simulink model "simulinkOSC_test"  (R2018b)
settings: Solver=FixedStepDiscrete  StartTime=0.0  StopTime=inf  FixedStep=0.01  RelTol=1e-3  EnableMultiTasking=on
model workspace (MAT data in the model file):
  gtest = 0
settings Model: Creator=Ulysses  LastModifiedBy=Ulysses
settings DataIOCC: LimitDataPoints=on  SaveFormat=Array
settings OptimizationCC: LifeSpan=inf
settings DebuggingCC: SolverPrmCheckMsg=warning  AllowSymbolicDim=off  SFUnexpectedBacktrackingDiag=warning  SFNoUnconditionalDefaultTransitionDiag=warning
settings HardwareCC: ProdBitPerPointer=32  ProdBitPerSizeT=32  ProdBitPerPtrDiffT=32  ProdLargestAtomicFloat=None  ProdIntDivRoundTo=Undefined  ProdEndianess=Unspecified  ProdWordSize=32  ProdHWDeviceType=32-bit Generic
settings ModelReferenceCC: PropagateSignalLabelsOutOfModel=off
settings SFSimCC: SimUseLocalCustomCode=off
settings RTWCC: RTWUseLocalCustomCode=off  TargetLang=C++
settings CodeAppCC: StateflowObjectComments=on
settings GRTTargetCC: TargetLangStandard=C89/C90 (ANSI)  GeneratePreprocessorConditionals=Disable all  MultiInstanceERTCode=on  CodeInterfacePackaging=C++ class
settings ConfigComp: CovMetricSettings=dw  CovHtmlReporting=on  CovSaveCumulativeToWorkspaceVar=on  CovSaveSingleToWorkspaceVar=on  CovExternalEMLEnable=off  CovSFcnEnable=off

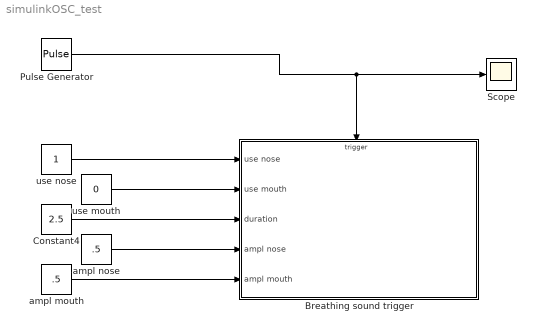
== system simulinkOSC_test ==
  Breathing sound trigger : Subsystem
  Constant4 : Constant  Value=2.5
  Pulse Generator : DiscretePulseGenerator  PulseType=Time based  Period=20000  PulseWidth=50
  Scope : Scope
  ampl mouth : Constant  Value=.5
  ampl nose : Constant  Value=.5
  use mouth : Constant  Value=0
  use nose : Constant
  wires:
  Constant4/1 -> Breathing sound trigger/3(duration)
  use nose/1 -> Breathing sound trigger/1(use nose)
  use mouth/1 -> Breathing sound trigger/2(use mouth)
  ampl nose/1 -> Breathing sound trigger/4(ampl nose)
  ampl mouth/1 -> Breathing sound trigger/5(ampl mouth)
  Pulse Generator/1 -> Breathing sound trigger/Trigger, Scope/1

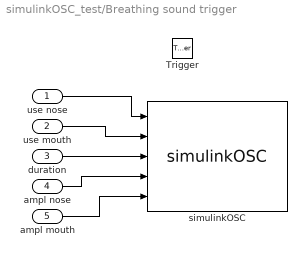
== system simulinkOSC_test/Breathing sound trigger ==
  use nose : Inport
  use mouth : Inport  Port=2
  duration : Inport  Port=3
  ampl nose : Inport  Port=4
  ampl mouth : Inport  Port=5
  Trigger : TriggerPort  VariantControl=Variant  PortDimensions=1
  simulinkOSC : S-Function  FunctionName=simulinkOSC  Parameters=uint16(server), uint16(port), uint16(pathsyndefs), uint16(pathwavs)  SFunctionDeploymentMode=off  EnableBusSupport=off  mask{server='localhost', port=57120, pathsyndefs='C:\\Users\\Ulysses\\Dropbox\\+SH_Projects\\VH_Breathing_Relaxation.git\\BreathingSound\\synthdefs', pathwavs='C:\\Users\\Ulysses\\Dropbox\\+SH_Projects\\VH_Breathing_Relaxation.git\\BreathingSound\\BrthSnd'}
      mask prompts: pathsyndefs "Path syndefs"; pathwavs "Path wavs"
      mask Display:
      | port_label('input', 1, 'use nose')
      | port_label('input', 2, 'use mouth')
      | port_label('input', 3, 'duration')
      | port_label('input', 4, 'ampl nose')
      | port_label('input', 5, 'ampl mouth')
  wires:
  duration/1 -> simulinkOSC/3
  ampl mouth/1 -> simulinkOSC/5
  ampl nose/1 -> simulinkOSC/4
  use nose/1 -> simulinkOSC/1
  use mouth/1 -> simulinkOSC/2
